simulink model "iranpour_9819893"  (R2022a)
settings: Solver=VariableStepAuto  StartTime=0.0  StopTime=0.04  FixedStep=1e-3  RelTol=1e-3
libraries: simulink x1, spsSawtoothGeneratorLib x1, cstblocks x1
settings Model: Creator=98912  LastModifiedBy=ZahraIranpour
settings SolverCC: AlgebraicLoopSolver=TrustRegion
settings DebuggingCC: UnconnectedInputMsg=warning  UnconnectedOutputMsg=warning  UnconnectedLineMsg=warning  SFMachineParentedDataDiag=warning
settings RTWCC: DLArmComputeVersion=19.05

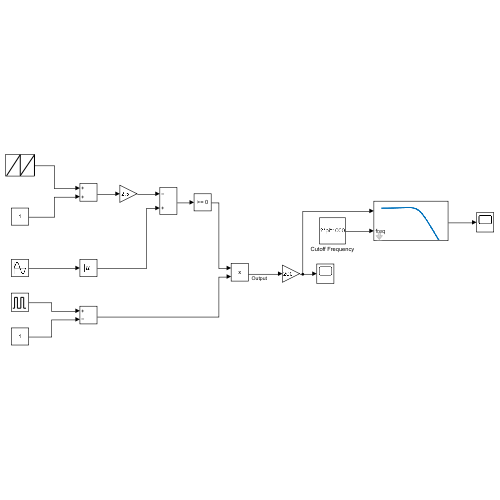
[thumbnail: Simulink's stored preview of the top-level diagram]
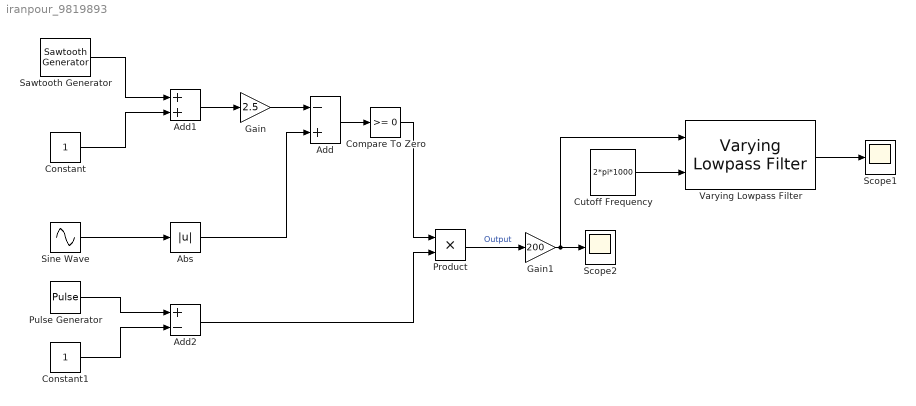
== system iranpour_9819893 ==
  Abs : Abs  SaturateOnIntegerOverflow=off
  Add : Sum  Inputs=-+
  Add1 : Sum
  Add2 : Sum  Inputs=+-
  Compare To Zero : simulink/Logic and Bit Operations/Compare To Zero  relop=>=  OutDataTypeStr=boolean
  Constant : Constant
  Constant1 : Constant
  Cutoff Frequency : Constant  Value=2*pi*1000
  Gain : Gain  Gain=2.5
  Gain1 : Gain  Gain=200
  Product : Product
  Pulse Generator : DiscretePulseGenerator  PulseType=Time based  Amplitude=2  Period=1/50  PulseWidth=50
  Sawtooth Generator : spsSawtoothGeneratorLib/Sawtooth Generator  Freq=20000  Phase=0  Ts=0
  Scope1 : Scope
  Scope2 : Scope
  Sine Wave : Sin  Amplitude=4  Frequency=2*pi*50  SampleTime=0
  Varying Lowpass Filter : cstblocks/Linear Parameter Varying/Varying Lowpass Filter  N=2
  wires:
  Add2/1 -> Product/2
  Sine Wave/1 -> Abs/1
  Add1/1 -> Gain/1
  Constant/1 -> Add1/2
  Constant1/1 -> Add2/2
  Gain/1 -> Add/1
  Pulse Generator/1 -> Add2/1
  Abs/1 -> Add/2
  Sawtooth Generator/1 -> Add1/1
  Add/1 -> Compare To Zero/1
  Product/1 -> Gain1/1  "Output"
  Compare To Zero/1 -> Product/1
  Gain1/1 -> Varying Lowpass Filter/1, Scope2/1
  Cutoff Frequency/1 -> Varying Lowpass Filter/2
  Varying Lowpass Filter/1 -> Scope1/1
